simulink model "mu_analysis_validation_model_with_modal_controller"  (R2020b)
settings: Solver=VariableStepAuto  StartTime=0.0  StopTime=200  RelTol=1e-3
values from neighbouring files (symbols this model uses):
  COUPLING_COEFFICIENT = 0.5736    [Workshop_MATLAB.m]
  ESTIMATOR_TRANSFER_FUNCTION_DENOMINATOR = [ESTIMATOR_TIME_CONSTANT 1]    [Workshop_MATLAB.m]
  ESTIMATOR_TRANSFER_FUNCTION_NUMERATOR = [1 0]    [Workshop_MATLAB.m]
  flexibleModeDampingRatioNominalValue = FLEXIBLE_MODE_DAMPING_RATIO    (= 0.00495)    [Workshop_MATLAB.m]
  flexibleModeFrequencyNominalValue = FLEXIBLE_MODE_FREQUENCY    (= 2.6268)    [Workshop_MATLAB.m]
  INITIAL_CONDITION_ON_STATE = 0.0001    [Workshop_MATLAB.m]
  satelliteInertiaNominalValue = SATELLITE_INERTIA    (= 31.38)    [Workshop_MATLAB.m]
  simulationModalGainMatrixStateFeedback = [0.517368537052283,6.148270360361254]    [Workshop_MATLAB.m]
undefined symbols (not defined in the file or in its folder): REACTION_WHEEL_REDUCED_FORM
settings Model: Creator=WLCG  LastModifiedBy=WLCG

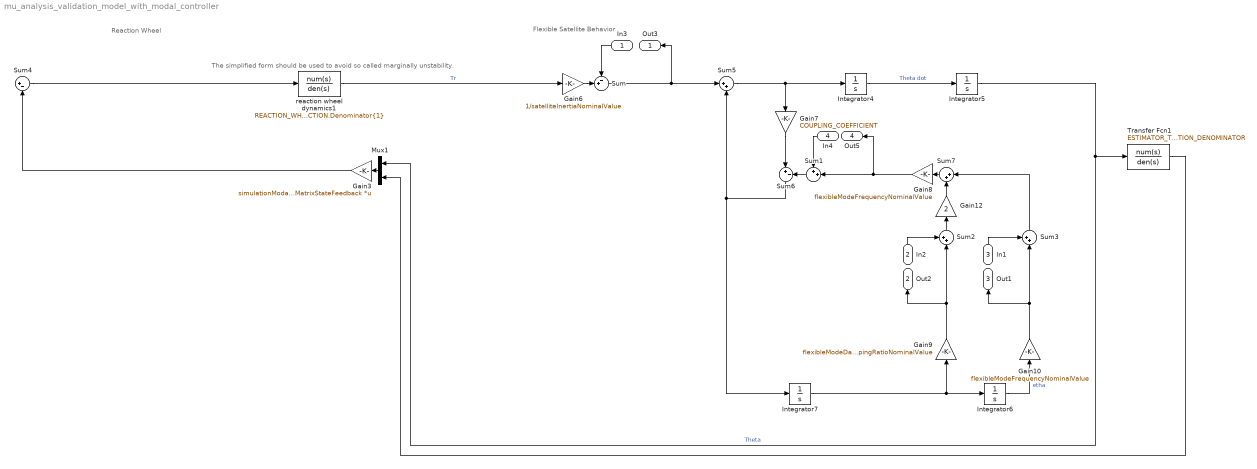
== system mu_analysis_validation_model_with_modal_controller ==
  note: Reaction Wheel
  note: Flexible Satellite Behavior
  note: The simplified form should be used to avoid so called marginally unstability.
  In3 : Inport
  In2 : Inport  Port=2
  In1 : Inport  Port=3
  In4 : Inport  Port=4
  Gain10 : Gain  Gain=flexibleModeFrequencyNominalValue
  Gain12 : Gain  Gain=2
  Gain3 : Gain  Gain=simulationModalGainMatrixStateFeedback  Multiplication=Matrix(K*u)
  Gain6 : Gain  Gain=1/satelliteInertiaNominalValue
  Gain7 : Gain  Gain=COUPLING_COEFFICIENT
  Gain8 : Gain  Gain=flexibleModeFrequencyNominalValue
  Gain9 : Gain  Gain=flexibleModeDampingRatioNominalValue
  Integrator4 : Integrator
  Integrator5 : Integrator
  Integrator6 : Integrator  InitialCondition=INITIAL_CONDITION_ON_STATE
  Integrator7 : Integrator
  Mux1 : Mux  Inputs=2
  Sum : Sum  Inputs=-+|
  Sum1 : Sum  Inputs=++|
  Sum2 : Sum  Inputs=++|
  Sum3 : Sum  Inputs=++|
  Sum4 : Sum  Inputs=|+-
  Sum5 : Sum  Inputs=|++
  Sum6 : Sum  Inputs=|+-
  Sum7 : Sum  Inputs=|++
  Transfer Fcn1 : TransferFcn  Numerator=ESTIMATOR_TRANSFER_FUNCTION_NUMERATOR  Denominator=ESTIMATOR_TRANSFER_FUNCTION_DENOMINATOR
  reaction wheel dynamics1 : TransferFcn  Numerator=REACTION_WHEEL_REDUCED_FORM.TRANSFER_FUNCTION.Numerator{1}  Denominator=REACTION_WHEEL_REDUCED_FORM.TRANSFER_FUNCTION.Denominator{1}
  Out3 : Outport
  Out2 : Outport  Port=2
  Out1 : Outport  Port=3
  Out5 : Outport  Port=4
  wires:
  Sum1/1 -> Sum6/2
  Sum6/1 -> Sum5/2, Integrator7/1
  Integrator7/1 -> Integrator6/1, Gain9/1
  reaction wheel dynamics1/1 -> Gain6/1  "Tr"
  Sum2/1 -> Gain12/1
  Integrator4/1 -> Integrator5/1  "Theta dot"
  Sum5/1 -> Gain7/1, Integrator4/1
  Sum7/1 -> Gain8/1
  Gain7/1 -> Sum6/1
  Gain6/1 -> Sum/2
  Sum3/1 -> Sum7/1
  Integrator6/1 -> Gain10/1  "etha"
  Gain12/1 -> Sum7/2
  Sum/1 -> Out3/1, Sum5/1
  Integrator5/1 -> Transfer Fcn1/1, Mux1/1  "Theta"
  Transfer Fcn1/1 -> Mux1/2
  Mux1/1 -> Gain3/1
  Gain8/1 -> Out5/1, Sum1/2
  In2/1 -> Sum2/1
  In1/1 -> Sum3/1
  In4/1 -> Sum1/1
  In3/1 -> Sum/1
  Gain9/1 -> Out2/1, Sum2/2
  Gain10/1 -> Out1/1, Sum3/2
  Gain3/1 -> Sum4/2
  Sum4/1 -> reaction wheel dynamics1/1
